simulink model "task1_lqr"  (R2021b)
settings: Solver=FixedStepAuto  StartTime=0.0  StopTime=1000  FixedStep=0.005  RelTol=1e-3
undefined symbols (not defined in the file): A, B, K1, K2, K3, Q1, Q2, Q3, R1, R2, R3, x0
settings Model: Creator=den  LastModifiedBy=den

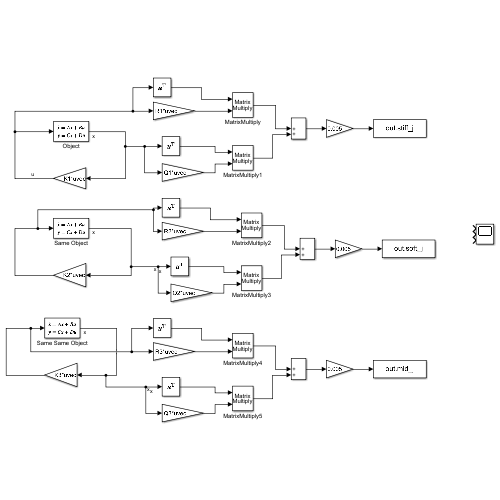
[thumbnail: Simulink's stored preview of the top-level diagram]
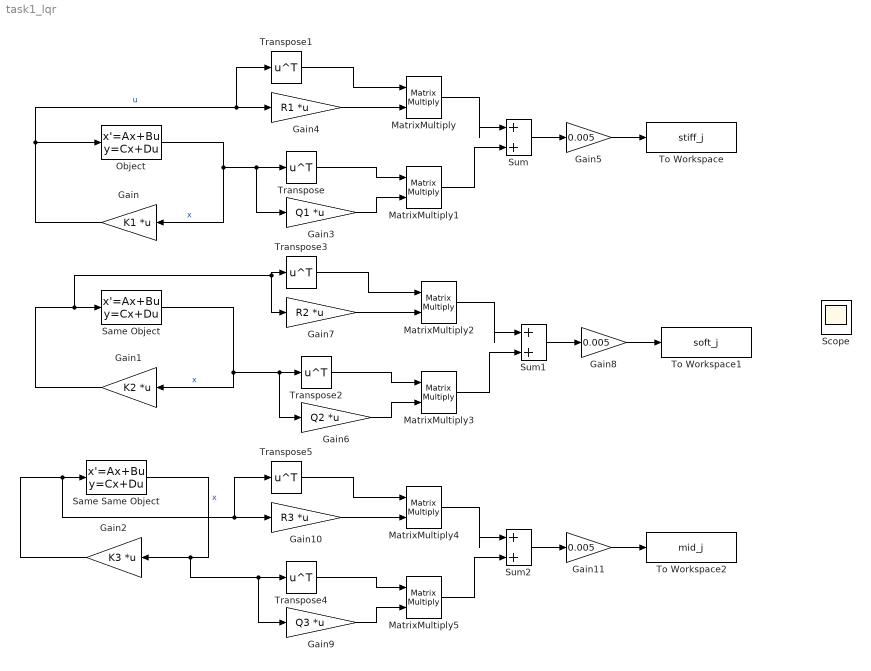
== system task1_lqr ==
  Gain : Gain  Gain=K1  Multiplication=Matrix(K*u) (u vector)
  Gain1 : Gain  Gain=K2  Multiplication=Matrix(K*u) (u vector)
  Gain10 : Gain  Gain=R3  Multiplication=Matrix(K*u) (u vector)
  Gain11 : Gain  Gain=0.005
  Gain2 : Gain  Gain=K3  Multiplication=Matrix(K*u) (u vector)
  Gain3 : Gain  Gain=Q1  Multiplication=Matrix(K*u) (u vector)
  Gain4 : Gain  Gain=R1  Multiplication=Matrix(K*u) (u vector)
  Gain5 : Gain  Gain=0.005
  Gain6 : Gain  Gain=Q2  Multiplication=Matrix(K*u) (u vector)
  Gain7 : Gain  Gain=R2  Multiplication=Matrix(K*u) (u vector)
  Gain8 : Gain  Gain=0.005
  Gain9 : Gain  Gain=Q3  Multiplication=Matrix(K*u) (u vector)
  MatrixMultiply{,1..5} (6 alike) : Product  Multiplication=Matrix(*)
  Object : StateSpace  A=A  B=B  C=[1 0 0 0; 0 1 0 0; 0 0 1 0; 0 0 0 1]  D=[0 0; 0 0; 0 0; 0 0]  InitialCondition=x0
  Same Object : StateSpace  A=A  B=B  C=[1 0 0 0; 0 1 0 0; 0 0 1 0; 0 0 0 1]  D=[0 0; 0 0; 0 0; 0 0]  InitialCondition=x0
  Same Same Object : StateSpace  A=A  B=B  C=[1 0 0 0; 0 1 0 0; 0 0 1 0; 0 0 0 1]  D=[0 0; 0 0; 0 0; 0 0]  InitialCondition=x0
  Scope : Scope  NumInputPorts=3
  Sum : Sum  Inputs=|++
  Sum1 : Sum  Inputs=|++
  Sum2 : Sum  Inputs=|++
  To Workspace : ToWorkspace  VariableName=stiff_j  SampleTime=-1
  To Workspace1 : ToWorkspace  VariableName=soft_j  SampleTime=-1
  To Workspace2 : ToWorkspace  VariableName=mid_j  SampleTime=-1
  Transpose{,1..5} (6 alike) : Math  Operator=transpose  SaturateOnIntegerOverflow=on
  wires:
  Object/1 -> Gain/1, Gain3/1, Transpose/1  "x"
  Gain/1 -> Transpose1/1, Gain4/1, Object/1  "u"
  Gain1/1 -> Gain7/1, Transpose3/1, Same Object/1
  Transpose/1 -> MatrixMultiply1/1
  Transpose1/1 -> MatrixMultiply/1
  Gain4/1 -> MatrixMultiply/2
  Gain3/1 -> MatrixMultiply1/2
  MatrixMultiply/1 -> Sum/1
  MatrixMultiply1/1 -> Sum/2
  Sum/1 -> Gain5/1
  Gain5/1 -> To Workspace/1
  Gain7/1 -> MatrixMultiply2/2
  Gain6/1 -> MatrixMultiply3/2
  Transpose3/1 -> MatrixMultiply2/1
  Sum1/1 -> Gain8/1
  Transpose2/1 -> MatrixMultiply3/1
  MatrixMultiply2/1 -> Sum1/1
  Gain8/1 -> To Workspace1/1
  MatrixMultiply3/1 -> Sum1/2
  Same Object/1 -> Gain6/1, Transpose2/1, Gain1/1  "x"
  Same Same Object/1 -> Gain9/1, Transpose4/1, Gain2/1  "x"
  MatrixMultiply5/1 -> Sum2/2
  Gain11/1 -> To Workspace2/1
  MatrixMultiply4/1 -> Sum2/1
  Gain2/1 -> Transpose5/1, Gain10/1, Same Same Object/1
  Transpose5/1 -> MatrixMultiply4/1
  Sum2/1 -> Gain11/1
  Gain9/1 -> MatrixMultiply5/2
  Transpose4/1 -> MatrixMultiply5/1
  Gain10/1 -> MatrixMultiply4/2
